simulink model "Effectors_UltraStick120"  (R2016b)
settings: Solver=VariableStepAuto  StartTime=0.0  StopTime=10  FixedStep=SampleTime  RelTol=1e-3
libraries: Surf_Lib x6
settings Model: Creator=Paul Freeman  LastModifiedBy=rega0051
settings DataIOCC: SaveOutput=off  SaveState=on  SaveTime=off
settings OptimizationCC: ExpressionDepthLimit=2147483647  LifeSpan=inf
settings DebuggingCC: SignalInfNanChecking=warning  SaveWithParameterizedLinksMsg=none  UnderspecifiedInitializationDetection=Classic  MergeDetectMultiDrivingBlocksExec=none  CheckMatrixSingularityMsg=warning  UnnecessaryDatatypeConvMsg=warning  FcnCallInpInsideContextMsg=warning  UnconnectedInputMsg=none  UnconnectedOutputMsg=none  UnconnectedLineMsg=none  SFcnCompatibilityMsg=warning  UniqueDataStoreMsg=warning  StateNameClashWarn=warning  SFUnexpectedBacktrackingDiag=warning  SFNoUnconditionalDefaultTransitionDiag=warning  SFExecutionAtInitializationDiag=none
settings HardwareCC: ProdBitPerPointer=32  ProdBitPerSizeT=32  ProdBitPerPtrDiffT=32  ProdLargestAtomicFloat=None  ProdWordSize=32  ProdHWDeviceType=Custom Processor->Custom
settings GRTTargetCC: TargetLangStandard=C89/C90 (ANSI)  GeneratePreprocessorConditionals=Disable all  CombineOutputUpdateFcns=off  GRTInterface=on
settings ConfigComp: CovMetricSettings=dw  CovHtmlReporting=on  CovSaveCumulativeToWorkspaceVar=on  CovSaveSingleToWorkspaceVar=on  CovExternalEMLEnable=off  CovSFcnEnable=off

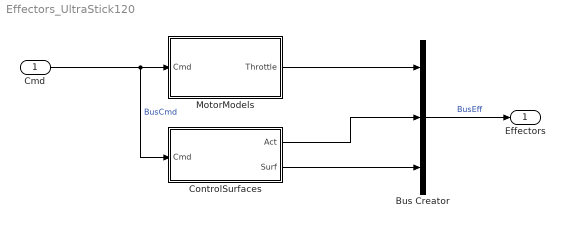
== system Effectors_UltraStick120 ==
  Cmd : Inport  OutDataTypeStr=Bus: BusCmd  SampleTime=0
  Bus Creator : BusCreator  Inputs=3  OutDataTypeStr=Bus: BusEff
      settings: AttributesFormatString=%<OutDataTypeStr>  InheritFromInputs=off
  ControlSurfaces : Subsystem
  MotorModels : Subsystem
  Effectors : Outport  OutDataTypeStr=Bus: BusEff  SampleTime=0
  wires:
  ControlSurfaces/1(Act) -> Bus Creator/2
  MotorModels/1(Throttle) -> Bus Creator/1
  Cmd/1 -> ControlSurfaces/1(Cmd), MotorModels/1(Cmd)  "BusCmd"
  ControlSurfaces/2(Surf) -> Bus Creator/3
  Bus Creator/1 -> Effectors/1  "BusEff"

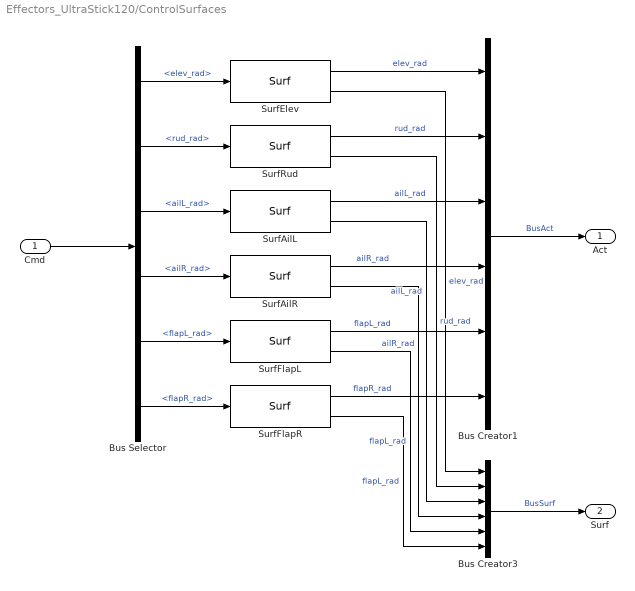
== system Effectors_UltraStick120/ControlSurfaces ==
  Cmd : Inport
  Bus Creator1 : BusCreator  Inputs=6  OutDataTypeStr=Bus: BusAct
      settings: AttributesFormatString=%<OutDataTypeStr>  InheritFromInputs=off
  Bus Creator3 : BusCreator  Inputs=6  OutDataTypeStr=Bus: BusSurf
      settings: AttributesFormatString=%<OutDataTypeStr>  InheritFromInputs=off
  Bus Selector : BusSelector  OutputSignals=elev_rad,rud_rad,ailL_rad,ailR_rad,flapL_rad,flapR_rad
  SurfAilL : Surf_Lib/Surf  surf=AC.Surf.ailL
  SurfAilR : Surf_Lib/Surf  surf=AC.Surf.ailR
  SurfElev : Surf_Lib/Surf  surf=AC.Surf.elev
  SurfFlapL : Surf_Lib/Surf  surf=AC.Surf.flapL
  SurfFlapR : Surf_Lib/Surf  surf=AC.Surf.flapR
  SurfRud : Surf_Lib/Surf  surf=AC.Surf.rud
  Act : Outport
  Surf : Outport  Port=2
  wires:
  SurfElev/1 -> Bus Creator1/1  "elev_rad"
  Bus Creator3/1 -> Surf/1  "BusSurf"
  SurfFlapR/2 -> Bus Creator3/6  "flapL_rad"
  SurfFlapL/2 -> Bus Creator3/5  "flapL_rad"
  SurfAilR/2 -> Bus Creator3/4  "ailR_rad"
  SurfAilL/2 -> Bus Creator3/3  "ailL_rad"
  SurfRud/2 -> Bus Creator3/2  "rud_rad"
  SurfElev/2 -> Bus Creator3/1  "elev_rad"
  Bus Selector/4 -> SurfAilR/1  "<ailR_rad>"
  SurfRud/1 -> Bus Creator1/2  "rud_rad"
  Bus Selector/6 -> SurfFlapR/1  "<flapR_rad>"
  SurfFlapR/1 -> Bus Creator1/6  "flapR_rad"
  SurfAilR/1 -> Bus Creator1/4  "ailR_rad"
  SurfFlapL/1 -> Bus Creator1/5  "flapL_rad"
  Bus Selector/5 -> SurfFlapL/1  "<flapL_rad>"
  SurfAilL/1 -> Bus Creator1/3  "ailL_rad"
  Bus Selector/3 -> SurfAilL/1  "<ailL_rad>"
  Bus Selector/2 -> SurfRud/1  "<rud_rad>"
  Bus Selector/1 -> SurfElev/1  "<elev_rad>"
  Cmd/1 -> Bus Selector/1
  Bus Creator1/1 -> Act/1  "BusAct"

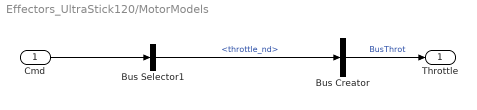
== system Effectors_UltraStick120/MotorModels ==
  Cmd : Inport  OutDataTypeStr=double
  Bus Creator : BusCreator  Inputs=1
  Bus Selector1 : BusSelector  OutputSignals=throttle_nd
  Throttle : Outport
  wires:
  Bus Creator/1 -> Throttle/1  "BusThrot"
  Bus Selector1/1 -> Bus Creator/1  "<throttle_nd>"
  Cmd/1 -> Bus Selector1/1
